simulink model "my_dom_trans"  (R2018a)
settings: Solver=VariableStepAuto  StartTime=0.0  StopTime=10000  RelTol=1e-3
values from neighbouring files (symbols this model uses):
  d_T_z = 0    [leveled_NL.m]    (also in leveled_state_space.m; leveled_transmitancja.m; my_dom.m; my_dom_state_space_script.m)
  d_T_zew = 0    [leveled_NL.m]    (also in leveled_state_space.m = 2; leveled_transmitancja.m = 2; my_dom.m; my_dom_state_space_script.m = 5)
  steptime = 1000    [leveled_NL.m]    (also in leveled_state_space.m; leveled_transmitancja.m; my_dom.m; my_dom_state_space_script.m)
  T_p1 = T_pN    (= 19)    [leveled_NL.m]    (also in leveled_state_space.m; leveled_transmitancja.m = 22; my_dom.m; my_dom_statyczne.m)
  T_wew1 = T_wewN    (= 21)    [leveled_NL.m]    (also in leveled_state_space.m; leveled_transmitancja.m = 27; my_dom.m; my_dom_statyczne.m)
undefined symbols (not defined in the file or in its folder): L1, L2, M1, M2
settings Model: Creator=johnb  LastModifiedBy=johnb

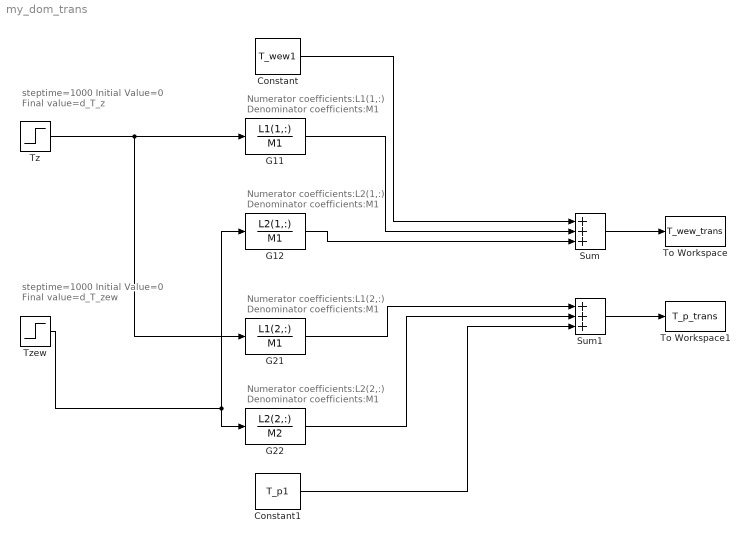
== system my_dom_trans ==
  note: Numerator coefficients:L1(1,:)
      | Denominator coefficients:M1
  note: steptime=1000
      | Initial Value=0
      | Final value=d_T_z
  note: steptime=1000
      | Initial Value=0
      | Final value=d_T_zew
  note: Numerator coefficients:L2(1,:)
      | Denominator coefficients:M1
  note: Numerator coefficients:L1(2,:)
      | Denominator coefficients:M1
  note: Numerator coefficients:L2(2,:)
      | Denominator coefficients:M1
  Constant : Constant  Value=T_wew1
  Constant1 : Constant  Value=T_p1
  G11 : TransferFcn  Numerator=L1(1,:)  Denominator=M1
  G12 : TransferFcn  Numerator=L2(1,:)  Denominator=M1
  G21 : TransferFcn  Numerator=L1(2,:)  Denominator=M1
  G22 : TransferFcn  Numerator=L2(2,:)  Denominator=M2
  Sum : Sum  Inputs=3
  Sum1 : Sum  Inputs=3
  To Workspace : ToWorkspace  VariableName=T_wew_trans  SaveFormat=Timeseries  SampleTime=-1
  To Workspace1 : ToWorkspace  VariableName=T_p_trans  SaveFormat=Timeseries  SampleTime=-1
  Tz : Step  Time=steptime  After=d_T_z  SampleTime=0
  "Tzew " : Step  Time=steptime  After=d_T_zew  SampleTime=0
  wires:
  Sum/1 -> To Workspace/1
  Sum1/1 -> To Workspace1/1
  Tz/1 -> G11/1, G21/1
  "Tzew "/1 -> G12/1, G22/1
  Constant/1 -> Sum/1
  G11/1 -> Sum/2
  G12/1 -> Sum/3
  G21/1 -> Sum1/1
  G22/1 -> Sum1/2
  Constant1/1 -> Sum1/3
